simulink model "Solar_MPPT_Inverter_Revived"  (R2020b)
settings: Solver=VariableStepAuto  StartTime=0.0  StopTime=1.5  RelTol=1e-3
libraries: powerlib x9, simulink x1, re_lib x1, powerlib_meascontrol x1
settings Model: Creator=amare  LastModifiedBy=amare

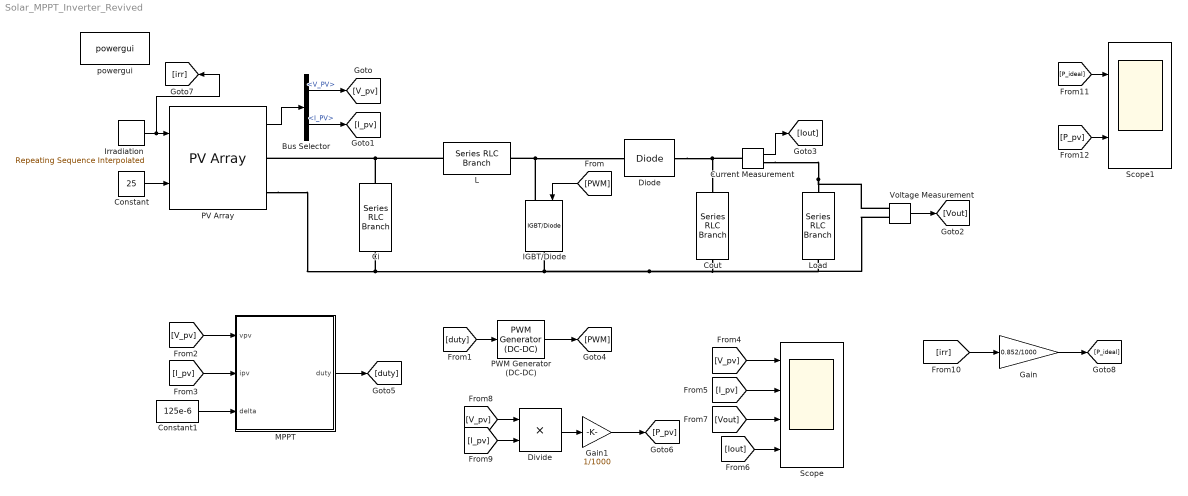
== system Solar_MPPT_Inverter_Revived ==
  Bus Selector : BusSelector  OutputSignals=V_PV,I_PV
  Ci : powerlib/Elements/Series RLC Branch  LConnTagsString=__new0  RConnTagsString=__new0  BranchType=RC  Resistance=1e-4  Inductance=1e-3  SetiL0=off  InitialCurrent=0  Capacitance=100e-6  Setx0=off  InitialVoltage=0  Measurements=None
  Constant : Constant  Value=25
  Constant1 : Constant  Value=125e-6
  Cout : powerlib/Elements/Series RLC Branch  LConnTagsString=__new0  RConnTagsString=__new0  BranchType=RC  Resistance=1e-4  Inductance=1e-3  SetiL0=off  InitialCurrent=0  Capacitance=100e-6  Setx0=off  InitialVoltage=0  Measurements=None
  Current Measurement : powerlib/Measurements/Current Measurement  PhasorSimulation=off  OutputType=Complex  PSBequivalent=0
  Diode : powerlib/Power Electronics/Diode  Ron=0.001  Lon=0  Vf=0.8  IC=0  UseSnubber=0  Rs=500  Cs=250e-9  Measurements=off
  Divide : Product  Inputs=**
  Gain : Gain  Gain=0.852/1000
  Gain1 : Gain  Gain=1/1000
  IGBT/Diode : powerlib/Power Electronics/IGBT//Diode  Ron=1e-3  Rs=1e5  Cs=inf  Measurements=off
  Irradiation : simulink/Sources/Repeating Sequence Interpolated  OutValues=[0 0 300 300 500 500 1000 1000 500 500 0 0].'  TimeValues=[0 0.25 0.2501 0.5 0.501 0.75 0.7501 1 1.01 1.25 1.2501 1.5].'  LookUpMeth=Interpolation-Use End Values  tsamp=0.01  OutMin=[]  OutMax=[]  OutDataTypeStr=double  OutputDataTypeScalingMode=double  OutDataType=fixdt(0,8)  OutScaling=2^-10
  L : powerlib/Elements/Series RLC Branch  LConnTagsString=__new0  RConnTagsString=__new0  BranchType=RL  Resistance=0.1  Inductance=2e-3  SetiL0=off  InitialCurrent=0  Capacitance=100e-6  Setx0=off  InitialVoltage=0  Measurements=None
  Load : powerlib/Elements/Series RLC Branch  LConnTagsString=__new0  RConnTagsString=__new0  BranchType=R  Resistance=20  Inductance=1e-3  SetiL0=off  InitialCurrent=0  Capacitance=100e-6  Setx0=off  InitialVoltage=0  Measurements=None
  MPPT : MATLAB Function  TreatAsAtomicUnit=on
  "PV Array " : re_lib/Solar/PV Array  Npar=2  Nser=2  PlotType=array @ 25 deg.C & specified irradiances  S_vec="[ 1000  500  100 ]"  Temp_C_vec="[ 45 25  ]"  ModuleName=User-defined  PlotWhenSelected=off  Pm=213.15  Ncell=60  Voc=36.3  Isc=7.84  Vm=29  Im=7.35  beta_Voc_pc=-0.36099  alpha_Isc_pc=0.102  beta_Voc=-0.13104  alpha_Isc=0.0079968  IL=7.8654  I0=2.9273e-10  nI=0.98119  Rsh=313.0553  Rs=0.39381  RobustModel=off  RobustCellTemperature=313.3991  BAL=on  Tc=1e-6  Tfilter=5e-5
  "PWM Generator (DC-DC) " : powerlib_meascontrol/Pulse & Signal Generators/PWM Generator (DC-DC)  Fsw=5000  Ts=5e-6
  Scope : Scope  NumInputPorts=4
  Scope1 : Scope  NumInputPorts=2
  Voltage Measurement : powerlib/Measurements/Voltage Measurement  PhasorSimulation=off  OutputType=Complex  PSBequivalent=0
  powergui : powerlib/powergui  Priority=1  SimulationMode=Discrete  SampleTime=5e-6  frequency=60  Iterations=50  frequencyindice=0  Pbase=100e6  ErrMax=1e-4  UnitsV=kV  UnitsW=MW  buscounter=0  FunctionMessages=off  echomessages=off  EnableUseOfTLC=off  CurrentSourceSwitches=off  DisableSnubberDevices=off  DisableRonSwitches=off  DisableVfSwitches=off  DisplayEquations=off  AutomaticDiscreteSolvers=off  SolverType=Tustin/Backward Euler (TBE)  Interpol=off  ExternalGateDelay=off  methode=off  Ts=100  x0status=blocks  SPID=on  SwTol=0  HookPort=off  NonlinearTolerance=1e-4  nMaxIteration=100  ContinueOnMaxIteration=off  RestoreLinks=warning  ResistiveCurrentMeasurement=off  Frange=[0:2:500]  Ylog=off  Xlog=on  ShowGrid=off  save=off  variable=ZData  structure=0  ZoomFFT=off  StartTime=0.0  cycles=1  DisplayStyle=1  fundamental=60  FreqAxis=off  MaxFrequency=1000  frequencyindicesteady=1  RmsSteady=1  display=off
  wires:
  Constant/1 -> "PV Array "/2
  Irradiation/1 -> [irr], "PV Array "/1
  "PV Array "/1 -> Bus Selector/1
  Bus Selector/2 -> [I_pv]  "<I_PV>"
  Bus Selector/1 -> [V_pv]  "<V_PV>"
  Current Measurement/1 -> [Iout]
  Voltage Measurement/1 -> [Vout]
  [duty] -> "PWM Generator (DC-DC) "/1
  [V_pv] -> MPPT/1(vpv)
  [I_pv] -> MPPT/2(ipv)
  Constant1/1 -> MPPT/3(delta)
  MPPT/1(duty) -> [duty]
  [V_pv] -> Scope/1
  [I_pv] -> Scope/2
  [Vout] -> Scope/3
  [Iout] -> Scope/4
  [V_pv] -> Divide/1
  [I_pv] -> Divide/2
  Divide/1 -> Gain1/1
  [irr] -> Gain/1
  "PWM Generator (DC-DC) "/1 -> [PWM]
  Gain/1 -> [P_ideal]
  [P_ideal] -> Scope1/1
  [P_pv] -> Scope1/2
  Gain1/1 -> [P_pv]
  [PWM] -> IGBT/Diode/1
  connections:
  Ci/LConn1 -- L/LConn1 -- "PV Array "/RConn1
  "PV Array "/RConn2 -- Voltage Measurement/LConn2 -- Load/RConn1 -- Cout/RConn1 -- IGBT/Diode/RConn1 -- Ci/RConn1
  IGBT/Diode/LConn1 -- Diode/LConn1 -- L/RConn1
  Diode/RConn1 -- Current Measurement/LConn1 -- Cout/LConn1
  Current Measurement/RConn1 -- Voltage Measurement/LConn1 -- Load/LConn1

== matlab function Solar_MPPT_Inverter_Revived/MPPT ==
  data: vpv input; duty output; ipv input; delta input
function duty = MPPT_algorithm(vpv,ipv,delta)
duty_init = 0.1;
duty_min=0; 
duty_max=0.85;

persistent Vold Pold duty_old;
if isempty(Vold)
    Vold=0;
    Pold=0;
    duty_old=duty_init;
end
P= vpv*ipv;
dV= vpv - Vold;
dP= P - Pold;

if dP ~=0 && vpv>30
    if dP < 0
        if dV < 0
            duty = duty_old - delta;
        else
            duty = duty_old + delta;
        end
    else
        if dV < 0
            duty = duty_old + delta;
        else
            duty = duty_old - delta;
        end
    end
else
    duty= duty_old;
end
if duty>=duty_max
    duty=duty_max;
elseif duty<duty_min
    duty=duty_min;
end

duty_old=duty;
Vold=vpv;
Pold=P;
